simulink model "gm_parallel_lht"  (R2019b)
settings: Solver=FixedStepDiscrete  StartTime=0.0  StopTime=inf  RelTol=1e-3
undefined symbols (not defined in the file or in its folder): bt, height, width
libraries: hdlsllib x190, simulink x13, hdlmdlgenlib x7, dspsrcs4 x1
(part 9 of 18)

== system gm_parallel_lht/Parallel LHT/Parallel LHT Accumulator/Accumulator with Switches/Accumulator_instance1/Block RAM ==
  wr_data : Inport  OutDataTypeStr=fixdt(0, 12, 0)  PortDimensions=1  SampleTime=6.66666666666667e-09
  wr_addr : Inport  Port=2  OutDataTypeStr=fixdt(0, 12, 0)  PortDimensions=1  SampleTime=6.66666666666667e-09
  wr_en : Inport  Port=3  OutDataTypeStr=boolean  PortDimensions=1  SampleTime=6.66666666666667e-09
  rd_addr : Inport  Port=4  OutDataTypeStr=fixdt(0, 12, 0)  PortDimensions=1  SampleTime=6.66666666666667e-09
  Simple Dual Port RAM : Subsystem
  rd_data : Outport
  wires:
  Simple Dual Port RAM/1(rd_data) -> rd_data/1
  wr_data/1 -> Simple Dual Port RAM/1(wr_data)
  wr_addr/1 -> Simple Dual Port RAM/2(wr_addr)
  wr_en/1 -> Simple Dual Port RAM/3(wr_en)
  rd_addr/1 -> Simple Dual Port RAM/4(rd_addr)

== system gm_parallel_lht/Parallel LHT/Parallel LHT Accumulator/Accumulator with Switches/Accumulator_instance10/Block RAM ==
  wr_data : Inport  OutDataTypeStr=fixdt(0, 12, 0)  PortDimensions=1  SampleTime=6.66666666666667e-09
  wr_addr : Inport  Port=2  OutDataTypeStr=fixdt(0, 12, 0)  PortDimensions=1  SampleTime=6.66666666666667e-09
  wr_en : Inport  Port=3  OutDataTypeStr=boolean  PortDimensions=1  SampleTime=6.66666666666667e-09
  rd_addr : Inport  Port=4  OutDataTypeStr=fixdt(0, 12, 0)  PortDimensions=1  SampleTime=6.66666666666667e-09
  Simple Dual Port RAM : Subsystem
  rd_data : Outport
  wires:
  rd_addr/1 -> Simple Dual Port RAM/4(rd_addr)
  wr_en/1 -> Simple Dual Port RAM/3(wr_en)
  wr_addr/1 -> Simple Dual Port RAM/2(wr_addr)
  wr_data/1 -> Simple Dual Port RAM/1(wr_data)
  Simple Dual Port RAM/1(rd_data) -> rd_data/1

== system gm_parallel_lht/Parallel LHT/Parallel LHT Accumulator/Accumulator with Switches/Accumulator_instance100/Block RAM ==
  wr_data : Inport  OutDataTypeStr=fixdt(0, 12, 0)  PortDimensions=1  SampleTime=6.66666666666667e-09
  wr_addr : Inport  Port=2  OutDataTypeStr=fixdt(0, 12, 0)  PortDimensions=1  SampleTime=6.66666666666667e-09
  wr_en : Inport  Port=3  OutDataTypeStr=boolean  PortDimensions=1  SampleTime=6.66666666666667e-09
  rd_addr : Inport  Port=4  OutDataTypeStr=fixdt(0, 12, 0)  PortDimensions=1  SampleTime=6.66666666666667e-09
  Simple Dual Port RAM : Subsystem
  rd_data : Outport
  wires:
  rd_addr/1 -> Simple Dual Port RAM/4(rd_addr)
  wr_en/1 -> Simple Dual Port RAM/3(wr_en)
  wr_addr/1 -> Simple Dual Port RAM/2(wr_addr)
  wr_data/1 -> Simple Dual Port RAM/1(wr_data)
  Simple Dual Port RAM/1(rd_data) -> rd_data/1

== system gm_parallel_lht/Parallel LHT/Parallel LHT Accumulator/Accumulator with Switches/Accumulator_instance101/Block RAM ==
  wr_data : Inport  OutDataTypeStr=fixdt(0, 12, 0)  PortDimensions=1  SampleTime=6.66666666666667e-09
  wr_addr : Inport  Port=2  OutDataTypeStr=fixdt(0, 12, 0)  PortDimensions=1  SampleTime=6.66666666666667e-09
  wr_en : Inport  Port=3  OutDataTypeStr=boolean  PortDimensions=1  SampleTime=6.66666666666667e-09
  rd_addr : Inport  Port=4  OutDataTypeStr=fixdt(0, 12, 0)  PortDimensions=1  SampleTime=6.66666666666667e-09
  Simple Dual Port RAM : Subsystem
  rd_data : Outport
  wires:
  rd_addr/1 -> Simple Dual Port RAM/4(rd_addr)
  wr_en/1 -> Simple Dual Port RAM/3(wr_en)
  wr_addr/1 -> Simple Dual Port RAM/2(wr_addr)
  wr_data/1 -> Simple Dual Port RAM/1(wr_data)
  Simple Dual Port RAM/1(rd_data) -> rd_data/1

== system gm_parallel_lht/Parallel LHT/Parallel LHT Accumulator/Accumulator with Switches/Accumulator_instance102/Block RAM ==
  wr_data : Inport  OutDataTypeStr=fixdt(0, 12, 0)  PortDimensions=1  SampleTime=6.66666666666667e-09
  wr_addr : Inport  Port=2  OutDataTypeStr=fixdt(0, 12, 0)  PortDimensions=1  SampleTime=6.66666666666667e-09
  wr_en : Inport  Port=3  OutDataTypeStr=boolean  PortDimensions=1  SampleTime=6.66666666666667e-09
  rd_addr : Inport  Port=4  OutDataTypeStr=fixdt(0, 12, 0)  PortDimensions=1  SampleTime=6.66666666666667e-09
  Simple Dual Port RAM : Subsystem
  rd_data : Outport
  wires:
  rd_addr/1 -> Simple Dual Port RAM/4(rd_addr)
  wr_en/1 -> Simple Dual Port RAM/3(wr_en)
  wr_addr/1 -> Simple Dual Port RAM/2(wr_addr)
  wr_data/1 -> Simple Dual Port RAM/1(wr_data)
  Simple Dual Port RAM/1(rd_data) -> rd_data/1

== system gm_parallel_lht/Parallel LHT/Parallel LHT Accumulator/Accumulator with Switches/Accumulator_instance103/Block RAM ==
  wr_data : Inport  OutDataTypeStr=fixdt(0, 12, 0)  PortDimensions=1  SampleTime=6.66666666666667e-09
  wr_addr : Inport  Port=2  OutDataTypeStr=fixdt(0, 12, 0)  PortDimensions=1  SampleTime=6.66666666666667e-09
  wr_en : Inport  Port=3  OutDataTypeStr=boolean  PortDimensions=1  SampleTime=6.66666666666667e-09
  rd_addr : Inport  Port=4  OutDataTypeStr=fixdt(0, 12, 0)  PortDimensions=1  SampleTime=6.66666666666667e-09
  Simple Dual Port RAM : Subsystem
  rd_data : Outport
  wires:
  rd_addr/1 -> Simple Dual Port RAM/4(rd_addr)
  wr_en/1 -> Simple Dual Port RAM/3(wr_en)
  wr_addr/1 -> Simple Dual Port RAM/2(wr_addr)
  wr_data/1 -> Simple Dual Port RAM/1(wr_data)
  Simple Dual Port RAM/1(rd_data) -> rd_data/1

== system gm_parallel_lht/Parallel LHT/Parallel LHT Accumulator/Accumulator with Switches/Accumulator_instance104/Block RAM ==
  wr_data : Inport  OutDataTypeStr=fixdt(0, 12, 0)  PortDimensions=1  SampleTime=6.66666666666667e-09
  wr_addr : Inport  Port=2  OutDataTypeStr=fixdt(0, 12, 0)  PortDimensions=1  SampleTime=6.66666666666667e-09
  wr_en : Inport  Port=3  OutDataTypeStr=boolean  PortDimensions=1  SampleTime=6.66666666666667e-09
  rd_addr : Inport  Port=4  OutDataTypeStr=fixdt(0, 12, 0)  PortDimensions=1  SampleTime=6.66666666666667e-09
  Simple Dual Port RAM : Subsystem
  rd_data : Outport
  wires:
  rd_addr/1 -> Simple Dual Port RAM/4(rd_addr)
  wr_en/1 -> Simple Dual Port RAM/3(wr_en)
  wr_addr/1 -> Simple Dual Port RAM/2(wr_addr)
  wr_data/1 -> Simple Dual Port RAM/1(wr_data)
  Simple Dual Port RAM/1(rd_data) -> rd_data/1

== system gm_parallel_lht/Parallel LHT/Parallel LHT Accumulator/Accumulator with Switches/Accumulator_instance105/Block RAM ==
  wr_data : Inport  OutDataTypeStr=fixdt(0, 12, 0)  PortDimensions=1  SampleTime=6.66666666666667e-09
  wr_addr : Inport  Port=2  OutDataTypeStr=fixdt(0, 12, 0)  PortDimensions=1  SampleTime=6.66666666666667e-09
  wr_en : Inport  Port=3  OutDataTypeStr=boolean  PortDimensions=1  SampleTime=6.66666666666667e-09
  rd_addr : Inport  Port=4  OutDataTypeStr=fixdt(0, 12, 0)  PortDimensions=1  SampleTime=6.66666666666667e-09
  Simple Dual Port RAM : Subsystem
  rd_data : Outport
  wires:
  rd_addr/1 -> Simple Dual Port RAM/4(rd_addr)
  wr_en/1 -> Simple Dual Port RAM/3(wr_en)
  wr_addr/1 -> Simple Dual Port RAM/2(wr_addr)
  wr_data/1 -> Simple Dual Port RAM/1(wr_data)
  Simple Dual Port RAM/1(rd_data) -> rd_data/1

== system gm_parallel_lht/Parallel LHT/Parallel LHT Accumulator/Accumulator with Switches/Accumulator_instance106/Block RAM ==
  wr_data : Inport  OutDataTypeStr=fixdt(0, 12, 0)  PortDimensions=1  SampleTime=6.66666666666667e-09
  wr_addr : Inport  Port=2  OutDataTypeStr=fixdt(0, 12, 0)  PortDimensions=1  SampleTime=6.66666666666667e-09
  wr_en : Inport  Port=3  OutDataTypeStr=boolean  PortDimensions=1  SampleTime=6.66666666666667e-09
  rd_addr : Inport  Port=4  OutDataTypeStr=fixdt(0, 12, 0)  PortDimensions=1  SampleTime=6.66666666666667e-09
  Simple Dual Port RAM : Subsystem
  rd_data : Outport
  wires:
  rd_addr/1 -> Simple Dual Port RAM/4(rd_addr)
  wr_en/1 -> Simple Dual Port RAM/3(wr_en)
  wr_addr/1 -> Simple Dual Port RAM/2(wr_addr)
  wr_data/1 -> Simple Dual Port RAM/1(wr_data)
  Simple Dual Port RAM/1(rd_data) -> rd_data/1

== system gm_parallel_lht/Parallel LHT/Parallel LHT Accumulator/Accumulator with Switches/Accumulator_instance107/Block RAM ==
  wr_data : Inport  OutDataTypeStr=fixdt(0, 12, 0)  PortDimensions=1  SampleTime=6.66666666666667e-09
  wr_addr : Inport  Port=2  OutDataTypeStr=fixdt(0, 12, 0)  PortDimensions=1  SampleTime=6.66666666666667e-09
  wr_en : Inport  Port=3  OutDataTypeStr=boolean  PortDimensions=1  SampleTime=6.66666666666667e-09
  rd_addr : Inport  Port=4  OutDataTypeStr=fixdt(0, 12, 0)  PortDimensions=1  SampleTime=6.66666666666667e-09
  Simple Dual Port RAM : Subsystem
  rd_data : Outport
  wires:
  rd_addr/1 -> Simple Dual Port RAM/4(rd_addr)
  wr_en/1 -> Simple Dual Port RAM/3(wr_en)
  wr_addr/1 -> Simple Dual Port RAM/2(wr_addr)
  wr_data/1 -> Simple Dual Port RAM/1(wr_data)
  Simple Dual Port RAM/1(rd_data) -> rd_data/1

== system gm_parallel_lht/Parallel LHT/Parallel LHT Accumulator/Accumulator with Switches/Accumulator_instance108/Block RAM ==
  wr_data : Inport  OutDataTypeStr=fixdt(0, 12, 0)  PortDimensions=1  SampleTime=6.66666666666667e-09
  wr_addr : Inport  Port=2  OutDataTypeStr=fixdt(0, 12, 0)  PortDimensions=1  SampleTime=6.66666666666667e-09
  wr_en : Inport  Port=3  OutDataTypeStr=boolean  PortDimensions=1  SampleTime=6.66666666666667e-09
  rd_addr : Inport  Port=4  OutDataTypeStr=fixdt(0, 12, 0)  PortDimensions=1  SampleTime=6.66666666666667e-09
  Simple Dual Port RAM : Subsystem
  rd_data : Outport
  wires:
  rd_addr/1 -> Simple Dual Port RAM/4(rd_addr)
  wr_en/1 -> Simple Dual Port RAM/3(wr_en)
  wr_addr/1 -> Simple Dual Port RAM/2(wr_addr)
  wr_data/1 -> Simple Dual Port RAM/1(wr_data)
  Simple Dual Port RAM/1(rd_data) -> rd_data/1

== system gm_parallel_lht/Parallel LHT/Parallel LHT Accumulator/Accumulator with Switches/Accumulator_instance109/Block RAM ==
  wr_data : Inport  OutDataTypeStr=fixdt(0, 12, 0)  PortDimensions=1  SampleTime=6.66666666666667e-09
  wr_addr : Inport  Port=2  OutDataTypeStr=fixdt(0, 12, 0)  PortDimensions=1  SampleTime=6.66666666666667e-09
  wr_en : Inport  Port=3  OutDataTypeStr=boolean  PortDimensions=1  SampleTime=6.66666666666667e-09
  rd_addr : Inport  Port=4  OutDataTypeStr=fixdt(0, 12, 0)  PortDimensions=1  SampleTime=6.66666666666667e-09
  Simple Dual Port RAM : Subsystem
  rd_data : Outport
  wires:
  rd_addr/1 -> Simple Dual Port RAM/4(rd_addr)
  wr_en/1 -> Simple Dual Port RAM/3(wr_en)
  wr_addr/1 -> Simple Dual Port RAM/2(wr_addr)
  wr_data/1 -> Simple Dual Port RAM/1(wr_data)
  Simple Dual Port RAM/1(rd_data) -> rd_data/1

== system gm_parallel_lht/Parallel LHT/Parallel LHT Accumulator/Accumulator with Switches/Accumulator_instance11/Block RAM ==
  wr_data : Inport  OutDataTypeStr=fixdt(0, 12, 0)  PortDimensions=1  SampleTime=6.66666666666667e-09
  wr_addr : Inport  Port=2  OutDataTypeStr=fixdt(0, 12, 0)  PortDimensions=1  SampleTime=6.66666666666667e-09
  wr_en : Inport  Port=3  OutDataTypeStr=boolean  PortDimensions=1  SampleTime=6.66666666666667e-09
  rd_addr : Inport  Port=4  OutDataTypeStr=fixdt(0, 12, 0)  PortDimensions=1  SampleTime=6.66666666666667e-09
  Simple Dual Port RAM : Subsystem
  rd_data : Outport
  wires:
  rd_addr/1 -> Simple Dual Port RAM/4(rd_addr)
  wr_en/1 -> Simple Dual Port RAM/3(wr_en)
  wr_addr/1 -> Simple Dual Port RAM/2(wr_addr)
  wr_data/1 -> Simple Dual Port RAM/1(wr_data)
  Simple Dual Port RAM/1(rd_data) -> rd_data/1

== system gm_parallel_lht/Parallel LHT/Parallel LHT Accumulator/Accumulator with Switches/Accumulator_instance110/Block RAM ==
  wr_data : Inport  OutDataTypeStr=fixdt(0, 12, 0)  PortDimensions=1  SampleTime=6.66666666666667e-09
  wr_addr : Inport  Port=2  OutDataTypeStr=fixdt(0, 12, 0)  PortDimensions=1  SampleTime=6.66666666666667e-09
  wr_en : Inport  Port=3  OutDataTypeStr=boolean  PortDimensions=1  SampleTime=6.66666666666667e-09
  rd_addr : Inport  Port=4  OutDataTypeStr=fixdt(0, 12, 0)  PortDimensions=1  SampleTime=6.66666666666667e-09
  Simple Dual Port RAM : Subsystem
  rd_data : Outport
  wires:
  rd_addr/1 -> Simple Dual Port RAM/4(rd_addr)
  wr_en/1 -> Simple Dual Port RAM/3(wr_en)
  wr_addr/1 -> Simple Dual Port RAM/2(wr_addr)
  wr_data/1 -> Simple Dual Port RAM/1(wr_data)
  Simple Dual Port RAM/1(rd_data) -> rd_data/1

== system gm_parallel_lht/Parallel LHT/Parallel LHT Accumulator/Accumulator with Switches/Accumulator_instance111/Block RAM ==
  wr_data : Inport  OutDataTypeStr=fixdt(0, 12, 0)  PortDimensions=1  SampleTime=6.66666666666667e-09
  wr_addr : Inport  Port=2  OutDataTypeStr=fixdt(0, 12, 0)  PortDimensions=1  SampleTime=6.66666666666667e-09
  wr_en : Inport  Port=3  OutDataTypeStr=boolean  PortDimensions=1  SampleTime=6.66666666666667e-09
  rd_addr : Inport  Port=4  OutDataTypeStr=fixdt(0, 12, 0)  PortDimensions=1  SampleTime=6.66666666666667e-09
  Simple Dual Port RAM : Subsystem
  rd_data : Outport
  wires:
  rd_addr/1 -> Simple Dual Port RAM/4(rd_addr)
  wr_en/1 -> Simple Dual Port RAM/3(wr_en)
  wr_addr/1 -> Simple Dual Port RAM/2(wr_addr)
  wr_data/1 -> Simple Dual Port RAM/1(wr_data)
  Simple Dual Port RAM/1(rd_data) -> rd_data/1

== system gm_parallel_lht/Parallel LHT/Parallel LHT Accumulator/Accumulator with Switches/Accumulator_instance112/Block RAM ==
  wr_data : Inport  OutDataTypeStr=fixdt(0, 12, 0)  PortDimensions=1  SampleTime=6.66666666666667e-09
  wr_addr : Inport  Port=2  OutDataTypeStr=fixdt(0, 12, 0)  PortDimensions=1  SampleTime=6.66666666666667e-09
  wr_en : Inport  Port=3  OutDataTypeStr=boolean  PortDimensions=1  SampleTime=6.66666666666667e-09
  rd_addr : Inport  Port=4  OutDataTypeStr=fixdt(0, 12, 0)  PortDimensions=1  SampleTime=6.66666666666667e-09
  Simple Dual Port RAM : Subsystem
  rd_data : Outport
  wires:
  rd_addr/1 -> Simple Dual Port RAM/4(rd_addr)
  wr_en/1 -> Simple Dual Port RAM/3(wr_en)
  wr_addr/1 -> Simple Dual Port RAM/2(wr_addr)
  wr_data/1 -> Simple Dual Port RAM/1(wr_data)
  Simple Dual Port RAM/1(rd_data) -> rd_data/1

== system gm_parallel_lht/Parallel LHT/Parallel LHT Accumulator/Accumulator with Switches/Accumulator_instance113/Block RAM ==
  wr_data : Inport  OutDataTypeStr=fixdt(0, 12, 0)  PortDimensions=1  SampleTime=6.66666666666667e-09
  wr_addr : Inport  Port=2  OutDataTypeStr=fixdt(0, 12, 0)  PortDimensions=1  SampleTime=6.66666666666667e-09
  wr_en : Inport  Port=3  OutDataTypeStr=boolean  PortDimensions=1  SampleTime=6.66666666666667e-09
  rd_addr : Inport  Port=4  OutDataTypeStr=fixdt(0, 12, 0)  PortDimensions=1  SampleTime=6.66666666666667e-09
  Simple Dual Port RAM : Subsystem
  rd_data : Outport
  wires:
  rd_addr/1 -> Simple Dual Port RAM/4(rd_addr)
  wr_en/1 -> Simple Dual Port RAM/3(wr_en)
  wr_addr/1 -> Simple Dual Port RAM/2(wr_addr)
  wr_data/1 -> Simple Dual Port RAM/1(wr_data)
  Simple Dual Port RAM/1(rd_data) -> rd_data/1

== system gm_parallel_lht/Parallel LHT/Parallel LHT Accumulator/Accumulator with Switches/Accumulator_instance114/Block RAM ==
  wr_data : Inport  OutDataTypeStr=fixdt(0, 12, 0)  PortDimensions=1  SampleTime=6.66666666666667e-09
  wr_addr : Inport  Port=2  OutDataTypeStr=fixdt(0, 12, 0)  PortDimensions=1  SampleTime=6.66666666666667e-09
  wr_en : Inport  Port=3  OutDataTypeStr=boolean  PortDimensions=1  SampleTime=6.66666666666667e-09
  rd_addr : Inport  Port=4  OutDataTypeStr=fixdt(0, 12, 0)  PortDimensions=1  SampleTime=6.66666666666667e-09
  Simple Dual Port RAM : Subsystem
  rd_data : Outport
  wires:
  rd_addr/1 -> Simple Dual Port RAM/4(rd_addr)
  wr_en/1 -> Simple Dual Port RAM/3(wr_en)
  wr_addr/1 -> Simple Dual Port RAM/2(wr_addr)
  wr_data/1 -> Simple Dual Port RAM/1(wr_data)
  Simple Dual Port RAM/1(rd_data) -> rd_data/1

== system gm_parallel_lht/Parallel LHT/Parallel LHT Accumulator/Accumulator with Switches/Accumulator_instance115/Block RAM ==
  wr_data : Inport  OutDataTypeStr=fixdt(0, 12, 0)  PortDimensions=1  SampleTime=6.66666666666667e-09
  wr_addr : Inport  Port=2  OutDataTypeStr=fixdt(0, 12, 0)  PortDimensions=1  SampleTime=6.66666666666667e-09
  wr_en : Inport  Port=3  OutDataTypeStr=boolean  PortDimensions=1  SampleTime=6.66666666666667e-09
  rd_addr : Inport  Port=4  OutDataTypeStr=fixdt(0, 12, 0)  PortDimensions=1  SampleTime=6.66666666666667e-09
  Simple Dual Port RAM : Subsystem
  rd_data : Outport
  wires:
  rd_addr/1 -> Simple Dual Port RAM/4(rd_addr)
  wr_en/1 -> Simple Dual Port RAM/3(wr_en)
  wr_addr/1 -> Simple Dual Port RAM/2(wr_addr)
  wr_data/1 -> Simple Dual Port RAM/1(wr_data)
  Simple Dual Port RAM/1(rd_data) -> rd_data/1

== system gm_parallel_lht/Parallel LHT/Parallel LHT Accumulator/Accumulator with Switches/Accumulator_instance116/Block RAM ==
  wr_data : Inport  OutDataTypeStr=fixdt(0, 12, 0)  PortDimensions=1  SampleTime=6.66666666666667e-09
  wr_addr : Inport  Port=2  OutDataTypeStr=fixdt(0, 12, 0)  PortDimensions=1  SampleTime=6.66666666666667e-09
  wr_en : Inport  Port=3  OutDataTypeStr=boolean  PortDimensions=1  SampleTime=6.66666666666667e-09
  rd_addr : Inport  Port=4  OutDataTypeStr=fixdt(0, 12, 0)  PortDimensions=1  SampleTime=6.66666666666667e-09
  Simple Dual Port RAM : Subsystem
  rd_data : Outport
  wires:
  rd_addr/1 -> Simple Dual Port RAM/4(rd_addr)
  wr_en/1 -> Simple Dual Port RAM/3(wr_en)
  wr_addr/1 -> Simple Dual Port RAM/2(wr_addr)
  wr_data/1 -> Simple Dual Port RAM/1(wr_data)
  Simple Dual Port RAM/1(rd_data) -> rd_data/1

== system gm_parallel_lht/Parallel LHT/Parallel LHT Accumulator/Accumulator with Switches/Accumulator_instance117/Block RAM ==
  wr_data : Inport  OutDataTypeStr=fixdt(0, 12, 0)  PortDimensions=1  SampleTime=6.66666666666667e-09
  wr_addr : Inport  Port=2  OutDataTypeStr=fixdt(0, 12, 0)  PortDimensions=1  SampleTime=6.66666666666667e-09
  wr_en : Inport  Port=3  OutDataTypeStr=boolean  PortDimensions=1  SampleTime=6.66666666666667e-09
  rd_addr : Inport  Port=4  OutDataTypeStr=fixdt(0, 12, 0)  PortDimensions=1  SampleTime=6.66666666666667e-09
  Simple Dual Port RAM : Subsystem
  rd_data : Outport
  wires:
  rd_addr/1 -> Simple Dual Port RAM/4(rd_addr)
  wr_en/1 -> Simple Dual Port RAM/3(wr_en)
  wr_addr/1 -> Simple Dual Port RAM/2(wr_addr)
  wr_data/1 -> Simple Dual Port RAM/1(wr_data)
  Simple Dual Port RAM/1(rd_data) -> rd_data/1

== system gm_parallel_lht/Parallel LHT/Parallel LHT Accumulator/Accumulator with Switches/Accumulator_instance118/Block RAM ==
  wr_data : Inport  OutDataTypeStr=fixdt(0, 12, 0)  PortDimensions=1  SampleTime=6.66666666666667e-09
  wr_addr : Inport  Port=2  OutDataTypeStr=fixdt(0, 12, 0)  PortDimensions=1  SampleTime=6.66666666666667e-09
  wr_en : Inport  Port=3  OutDataTypeStr=boolean  PortDimensions=1  SampleTime=6.66666666666667e-09
  rd_addr : Inport  Port=4  OutDataTypeStr=fixdt(0, 12, 0)  PortDimensions=1  SampleTime=6.66666666666667e-09
  Simple Dual Port RAM : Subsystem
  rd_data : Outport
  wires:
  rd_addr/1 -> Simple Dual Port RAM/4(rd_addr)
  wr_en/1 -> Simple Dual Port RAM/3(wr_en)
  wr_addr/1 -> Simple Dual Port RAM/2(wr_addr)
  wr_data/1 -> Simple Dual Port RAM/1(wr_data)
  Simple Dual Port RAM/1(rd_data) -> rd_data/1

== system gm_parallel_lht/Parallel LHT/Parallel LHT Accumulator/Accumulator with Switches/Accumulator_instance119/Block RAM ==
  wr_data : Inport  OutDataTypeStr=fixdt(0, 12, 0)  PortDimensions=1  SampleTime=6.66666666666667e-09
  wr_addr : Inport  Port=2  OutDataTypeStr=fixdt(0, 12, 0)  PortDimensions=1  SampleTime=6.66666666666667e-09
  wr_en : Inport  Port=3  OutDataTypeStr=boolean  PortDimensions=1  SampleTime=6.66666666666667e-09
  rd_addr : Inport  Port=4  OutDataTypeStr=fixdt(0, 12, 0)  PortDimensions=1  SampleTime=6.66666666666667e-09
  Simple Dual Port RAM : Subsystem
  rd_data : Outport
  wires:
  rd_addr/1 -> Simple Dual Port RAM/4(rd_addr)
  wr_en/1 -> Simple Dual Port RAM/3(wr_en)
  wr_addr/1 -> Simple Dual Port RAM/2(wr_addr)
  wr_data/1 -> Simple Dual Port RAM/1(wr_data)
  Simple Dual Port RAM/1(rd_data) -> rd_data/1

== system gm_parallel_lht/Parallel LHT/Parallel LHT Accumulator/Accumulator with Switches/Accumulator_instance12/Block RAM ==
  wr_data : Inport  OutDataTypeStr=fixdt(0, 12, 0)  PortDimensions=1  SampleTime=6.66666666666667e-09
  wr_addr : Inport  Port=2  OutDataTypeStr=fixdt(0, 12, 0)  PortDimensions=1  SampleTime=6.66666666666667e-09
  wr_en : Inport  Port=3  OutDataTypeStr=boolean  PortDimensions=1  SampleTime=6.66666666666667e-09
  rd_addr : Inport  Port=4  OutDataTypeStr=fixdt(0, 12, 0)  PortDimensions=1  SampleTime=6.66666666666667e-09
  Simple Dual Port RAM : Subsystem
  rd_data : Outport
  wires:
  rd_addr/1 -> Simple Dual Port RAM/4(rd_addr)
  wr_en/1 -> Simple Dual Port RAM/3(wr_en)
  wr_addr/1 -> Simple Dual Port RAM/2(wr_addr)
  wr_data/1 -> Simple Dual Port RAM/1(wr_data)
  Simple Dual Port RAM/1(rd_data) -> rd_data/1

== system gm_parallel_lht/Parallel LHT/Parallel LHT Accumulator/Accumulator with Switches/Accumulator_instance120/Block RAM ==
  wr_data : Inport  OutDataTypeStr=fixdt(0, 12, 0)  PortDimensions=1  SampleTime=6.66666666666667e-09
  wr_addr : Inport  Port=2  OutDataTypeStr=fixdt(0, 12, 0)  PortDimensions=1  SampleTime=6.66666666666667e-09
  wr_en : Inport  Port=3  OutDataTypeStr=boolean  PortDimensions=1  SampleTime=6.66666666666667e-09
  rd_addr : Inport  Port=4  OutDataTypeStr=fixdt(0, 12, 0)  PortDimensions=1  SampleTime=6.66666666666667e-09
  Simple Dual Port RAM : Subsystem
  rd_data : Outport
  wires:
  rd_addr/1 -> Simple Dual Port RAM/4(rd_addr)
  wr_en/1 -> Simple Dual Port RAM/3(wr_en)
  wr_addr/1 -> Simple Dual Port RAM/2(wr_addr)
  wr_data/1 -> Simple Dual Port RAM/1(wr_data)
  Simple Dual Port RAM/1(rd_data) -> rd_data/1

== system gm_parallel_lht/Parallel LHT/Parallel LHT Accumulator/Accumulator with Switches/Accumulator_instance121/Block RAM ==
  wr_data : Inport  OutDataTypeStr=fixdt(0, 12, 0)  PortDimensions=1  SampleTime=6.66666666666667e-09
  wr_addr : Inport  Port=2  OutDataTypeStr=fixdt(0, 12, 0)  PortDimensions=1  SampleTime=6.66666666666667e-09
  wr_en : Inport  Port=3  OutDataTypeStr=boolean  PortDimensions=1  SampleTime=6.66666666666667e-09
  rd_addr : Inport  Port=4  OutDataTypeStr=fixdt(0, 12, 0)  PortDimensions=1  SampleTime=6.66666666666667e-09
  Simple Dual Port RAM : Subsystem
  rd_data : Outport
  wires:
  rd_addr/1 -> Simple Dual Port RAM/4(rd_addr)
  wr_en/1 -> Simple Dual Port RAM/3(wr_en)
  wr_addr/1 -> Simple Dual Port RAM/2(wr_addr)
  wr_data/1 -> Simple Dual Port RAM/1(wr_data)
  Simple Dual Port RAM/1(rd_data) -> rd_data/1

== system gm_parallel_lht/Parallel LHT/Parallel LHT Accumulator/Accumulator with Switches/Accumulator_instance122/Block RAM ==
  wr_data : Inport  OutDataTypeStr=fixdt(0, 12, 0)  PortDimensions=1  SampleTime=6.66666666666667e-09
  wr_addr : Inport  Port=2  OutDataTypeStr=fixdt(0, 12, 0)  PortDimensions=1  SampleTime=6.66666666666667e-09
  wr_en : Inport  Port=3  OutDataTypeStr=boolean  PortDimensions=1  SampleTime=6.66666666666667e-09
  rd_addr : Inport  Port=4  OutDataTypeStr=fixdt(0, 12, 0)  PortDimensions=1  SampleTime=6.66666666666667e-09
  Simple Dual Port RAM : Subsystem
  rd_data : Outport
  wires:
  rd_addr/1 -> Simple Dual Port RAM/4(rd_addr)
  wr_en/1 -> Simple Dual Port RAM/3(wr_en)
  wr_addr/1 -> Simple Dual Port RAM/2(wr_addr)
  wr_data/1 -> Simple Dual Port RAM/1(wr_data)
  Simple Dual Port RAM/1(rd_data) -> rd_data/1

== system gm_parallel_lht/Parallel LHT/Parallel LHT Accumulator/Accumulator with Switches/Accumulator_instance123/Block RAM ==
  wr_data : Inport  OutDataTypeStr=fixdt(0, 12, 0)  PortDimensions=1  SampleTime=6.66666666666667e-09
  wr_addr : Inport  Port=2  OutDataTypeStr=fixdt(0, 12, 0)  PortDimensions=1  SampleTime=6.66666666666667e-09
  wr_en : Inport  Port=3  OutDataTypeStr=boolean  PortDimensions=1  SampleTime=6.66666666666667e-09
  rd_addr : Inport  Port=4  OutDataTypeStr=fixdt(0, 12, 0)  PortDimensions=1  SampleTime=6.66666666666667e-09
  Simple Dual Port RAM : Subsystem
  rd_data : Outport
  wires:
  rd_addr/1 -> Simple Dual Port RAM/4(rd_addr)
  wr_en/1 -> Simple Dual Port RAM/3(wr_en)
  wr_addr/1 -> Simple Dual Port RAM/2(wr_addr)
  wr_data/1 -> Simple Dual Port RAM/1(wr_data)
  Simple Dual Port RAM/1(rd_data) -> rd_data/1

== system gm_parallel_lht/Parallel LHT/Parallel LHT Accumulator/Accumulator with Switches/Accumulator_instance124/Block RAM ==
  wr_data : Inport  OutDataTypeStr=fixdt(0, 12, 0)  PortDimensions=1  SampleTime=6.66666666666667e-09
  wr_addr : Inport  Port=2  OutDataTypeStr=fixdt(0, 12, 0)  PortDimensions=1  SampleTime=6.66666666666667e-09
  wr_en : Inport  Port=3  OutDataTypeStr=boolean  PortDimensions=1  SampleTime=6.66666666666667e-09
  rd_addr : Inport  Port=4  OutDataTypeStr=fixdt(0, 12, 0)  PortDimensions=1  SampleTime=6.66666666666667e-09
  Simple Dual Port RAM : Subsystem
  rd_data : Outport
  wires:
  rd_addr/1 -> Simple Dual Port RAM/4(rd_addr)
  wr_en/1 -> Simple Dual Port RAM/3(wr_en)
  wr_addr/1 -> Simple Dual Port RAM/2(wr_addr)
  wr_data/1 -> Simple Dual Port RAM/1(wr_data)
  Simple Dual Port RAM/1(rd_data) -> rd_data/1

== system gm_parallel_lht/Parallel LHT/Parallel LHT Accumulator/Accumulator with Switches/Accumulator_instance125/Block RAM ==
  wr_data : Inport  OutDataTypeStr=fixdt(0, 12, 0)  PortDimensions=1  SampleTime=6.66666666666667e-09
  wr_addr : Inport  Port=2  OutDataTypeStr=fixdt(0, 12, 0)  PortDimensions=1  SampleTime=6.66666666666667e-09
  wr_en : Inport  Port=3  OutDataTypeStr=boolean  PortDimensions=1  SampleTime=6.66666666666667e-09
  rd_addr : Inport  Port=4  OutDataTypeStr=fixdt(0, 12, 0)  PortDimensions=1  SampleTime=6.66666666666667e-09
  Simple Dual Port RAM : Subsystem
  rd_data : Outport
  wires:
  rd_addr/1 -> Simple Dual Port RAM/4(rd_addr)
  wr_en/1 -> Simple Dual Port RAM/3(wr_en)
  wr_addr/1 -> Simple Dual Port RAM/2(wr_addr)
  wr_data/1 -> Simple Dual Port RAM/1(wr_data)
  Simple Dual Port RAM/1(rd_data) -> rd_data/1

== system gm_parallel_lht/Parallel LHT/Parallel LHT Accumulator/Accumulator with Switches/Accumulator_instance126/Block RAM ==
  wr_data : Inport  OutDataTypeStr=fixdt(0, 12, 0)  PortDimensions=1  SampleTime=6.66666666666667e-09
  wr_addr : Inport  Port=2  OutDataTypeStr=fixdt(0, 12, 0)  PortDimensions=1  SampleTime=6.66666666666667e-09
  wr_en : Inport  Port=3  OutDataTypeStr=boolean  PortDimensions=1  SampleTime=6.66666666666667e-09
  rd_addr : Inport  Port=4  OutDataTypeStr=fixdt(0, 12, 0)  PortDimensions=1  SampleTime=6.66666666666667e-09
  Simple Dual Port RAM : Subsystem
  rd_data : Outport
  wires:
  rd_addr/1 -> Simple Dual Port RAM/4(rd_addr)
  wr_en/1 -> Simple Dual Port RAM/3(wr_en)
  wr_addr/1 -> Simple Dual Port RAM/2(wr_addr)
  wr_data/1 -> Simple Dual Port RAM/1(wr_data)
  Simple Dual Port RAM/1(rd_data) -> rd_data/1

== system gm_parallel_lht/Parallel LHT/Parallel LHT Accumulator/Accumulator with Switches/Accumulator_instance127/Block RAM ==
  wr_data : Inport  OutDataTypeStr=fixdt(0, 12, 0)  PortDimensions=1  SampleTime=6.66666666666667e-09
  wr_addr : Inport  Port=2  OutDataTypeStr=fixdt(0, 12, 0)  PortDimensions=1  SampleTime=6.66666666666667e-09
  wr_en : Inport  Port=3  OutDataTypeStr=boolean  PortDimensions=1  SampleTime=6.66666666666667e-09
  rd_addr : Inport  Port=4  OutDataTypeStr=fixdt(0, 12, 0)  PortDimensions=1  SampleTime=6.66666666666667e-09
  Simple Dual Port RAM : Subsystem
  rd_data : Outport
  wires:
  rd_addr/1 -> Simple Dual Port RAM/4(rd_addr)
  wr_en/1 -> Simple Dual Port RAM/3(wr_en)
  wr_addr/1 -> Simple Dual Port RAM/2(wr_addr)
  wr_data/1 -> Simple Dual Port RAM/1(wr_data)
  Simple Dual Port RAM/1(rd_data) -> rd_data/1

== system gm_parallel_lht/Parallel LHT/Parallel LHT Accumulator/Accumulator with Switches/Accumulator_instance128/Block RAM ==
  wr_data : Inport  OutDataTypeStr=fixdt(0, 12, 0)  PortDimensions=1  SampleTime=6.66666666666667e-09
  wr_addr : Inport  Port=2  OutDataTypeStr=fixdt(0, 12, 0)  PortDimensions=1  SampleTime=6.66666666666667e-09
  wr_en : Inport  Port=3  OutDataTypeStr=boolean  PortDimensions=1  SampleTime=6.66666666666667e-09
  rd_addr : Inport  Port=4  OutDataTypeStr=fixdt(0, 12, 0)  PortDimensions=1  SampleTime=6.66666666666667e-09
  Simple Dual Port RAM : Subsystem
  rd_data : Outport
  wires:
  rd_addr/1 -> Simple Dual Port RAM/4(rd_addr)
  wr_en/1 -> Simple Dual Port RAM/3(wr_en)
  wr_addr/1 -> Simple Dual Port RAM/2(wr_addr)
  wr_data/1 -> Simple Dual Port RAM/1(wr_data)
  Simple Dual Port RAM/1(rd_data) -> rd_data/1

== system gm_parallel_lht/Parallel LHT/Parallel LHT Accumulator/Accumulator with Switches/Accumulator_instance129/Block RAM ==
  wr_data : Inport  OutDataTypeStr=fixdt(0, 12, 0)  PortDimensions=1  SampleTime=6.66666666666667e-09
  wr_addr : Inport  Port=2  OutDataTypeStr=fixdt(0, 12, 0)  PortDimensions=1  SampleTime=6.66666666666667e-09
  wr_en : Inport  Port=3  OutDataTypeStr=boolean  PortDimensions=1  SampleTime=6.66666666666667e-09
  rd_addr : Inport  Port=4  OutDataTypeStr=fixdt(0, 12, 0)  PortDimensions=1  SampleTime=6.66666666666667e-09
  Simple Dual Port RAM : Subsystem
  rd_data : Outport
  wires:
  rd_addr/1 -> Simple Dual Port RAM/4(rd_addr)
  wr_en/1 -> Simple Dual Port RAM/3(wr_en)
  wr_addr/1 -> Simple Dual Port RAM/2(wr_addr)
  wr_data/1 -> Simple Dual Port RAM/1(wr_data)
  Simple Dual Port RAM/1(rd_data) -> rd_data/1

== system gm_parallel_lht/Parallel LHT/Parallel LHT Accumulator/Accumulator with Switches/Accumulator_instance13/Block RAM ==
  wr_data : Inport  OutDataTypeStr=fixdt(0, 12, 0)  PortDimensions=1  SampleTime=6.66666666666667e-09
  wr_addr : Inport  Port=2  OutDataTypeStr=fixdt(0, 12, 0)  PortDimensions=1  SampleTime=6.66666666666667e-09
  wr_en : Inport  Port=3  OutDataTypeStr=boolean  PortDimensions=1  SampleTime=6.66666666666667e-09
  rd_addr : Inport  Port=4  OutDataTypeStr=fixdt(0, 12, 0)  PortDimensions=1  SampleTime=6.66666666666667e-09
  Simple Dual Port RAM : Subsystem
  rd_data : Outport
  wires:
  rd_addr/1 -> Simple Dual Port RAM/4(rd_addr)
  wr_en/1 -> Simple Dual Port RAM/3(wr_en)
  wr_addr/1 -> Simple Dual Port RAM/2(wr_addr)
  wr_data/1 -> Simple Dual Port RAM/1(wr_data)
  Simple Dual Port RAM/1(rd_data) -> rd_data/1

== system gm_parallel_lht/Parallel LHT/Parallel LHT Accumulator/Accumulator with Switches/Accumulator_instance130/Block RAM ==
  wr_data : Inport  OutDataTypeStr=fixdt(0, 12, 0)  PortDimensions=1  SampleTime=6.66666666666667e-09
  wr_addr : Inport  Port=2  OutDataTypeStr=fixdt(0, 12, 0)  PortDimensions=1  SampleTime=6.66666666666667e-09
  wr_en : Inport  Port=3  OutDataTypeStr=boolean  PortDimensions=1  SampleTime=6.66666666666667e-09
  rd_addr : Inport  Port=4  OutDataTypeStr=fixdt(0, 12, 0)  PortDimensions=1  SampleTime=6.66666666666667e-09
  Simple Dual Port RAM : Subsystem
  rd_data : Outport
  wires:
  rd_addr/1 -> Simple Dual Port RAM/4(rd_addr)
  wr_en/1 -> Simple Dual Port RAM/3(wr_en)
  wr_addr/1 -> Simple Dual Port RAM/2(wr_addr)
  wr_data/1 -> Simple Dual Port RAM/1(wr_data)
  Simple Dual Port RAM/1(rd_data) -> rd_data/1

== system gm_parallel_lht/Parallel LHT/Parallel LHT Accumulator/Accumulator with Switches/Accumulator_instance131/Block RAM ==
  wr_data : Inport  OutDataTypeStr=fixdt(0, 12, 0)  PortDimensions=1  SampleTime=6.66666666666667e-09
  wr_addr : Inport  Port=2  OutDataTypeStr=fixdt(0, 12, 0)  PortDimensions=1  SampleTime=6.66666666666667e-09
  wr_en : Inport  Port=3  OutDataTypeStr=boolean  PortDimensions=1  SampleTime=6.66666666666667e-09
  rd_addr : Inport  Port=4  OutDataTypeStr=fixdt(0, 12, 0)  PortDimensions=1  SampleTime=6.66666666666667e-09
  Simple Dual Port RAM : Subsystem
  rd_data : Outport
  wires:
  rd_addr/1 -> Simple Dual Port RAM/4(rd_addr)
  wr_en/1 -> Simple Dual Port RAM/3(wr_en)
  wr_addr/1 -> Simple Dual Port RAM/2(wr_addr)
  wr_data/1 -> Simple Dual Port RAM/1(wr_data)
  Simple Dual Port RAM/1(rd_data) -> rd_data/1

== system gm_parallel_lht/Parallel LHT/Parallel LHT Accumulator/Accumulator with Switches/Accumulator_instance132/Block RAM ==
  wr_data : Inport  OutDataTypeStr=fixdt(0, 12, 0)  PortDimensions=1  SampleTime=6.66666666666667e-09
  wr_addr : Inport  Port=2  OutDataTypeStr=fixdt(0, 12, 0)  PortDimensions=1  SampleTime=6.66666666666667e-09
  wr_en : Inport  Port=3  OutDataTypeStr=boolean  PortDimensions=1  SampleTime=6.66666666666667e-09
  rd_addr : Inport  Port=4  OutDataTypeStr=fixdt(0, 12, 0)  PortDimensions=1  SampleTime=6.66666666666667e-09
  Simple Dual Port RAM : Subsystem
  rd_data : Outport
  wires:
  rd_addr/1 -> Simple Dual Port RAM/4(rd_addr)
  wr_en/1 -> Simple Dual Port RAM/3(wr_en)
  wr_addr/1 -> Simple Dual Port RAM/2(wr_addr)
  wr_data/1 -> Simple Dual Port RAM/1(wr_data)
  Simple Dual Port RAM/1(rd_data) -> rd_data/1

== system gm_parallel_lht/Parallel LHT/Parallel LHT Accumulator/Accumulator with Switches/Accumulator_instance133/Block RAM ==
  wr_data : Inport  OutDataTypeStr=fixdt(0, 12, 0)  PortDimensions=1  SampleTime=6.66666666666667e-09
  wr_addr : Inport  Port=2  OutDataTypeStr=fixdt(0, 12, 0)  PortDimensions=1  SampleTime=6.66666666666667e-09
  wr_en : Inport  Port=3  OutDataTypeStr=boolean  PortDimensions=1  SampleTime=6.66666666666667e-09
  rd_addr : Inport  Port=4  OutDataTypeStr=fixdt(0, 12, 0)  PortDimensions=1  SampleTime=6.66666666666667e-09
  Simple Dual Port RAM : Subsystem
  rd_data : Outport
  wires:
  rd_addr/1 -> Simple Dual Port RAM/4(rd_addr)
  wr_en/1 -> Simple Dual Port RAM/3(wr_en)
  wr_addr/1 -> Simple Dual Port RAM/2(wr_addr)
  wr_data/1 -> Simple Dual Port RAM/1(wr_data)
  Simple Dual Port RAM/1(rd_data) -> rd_data/1

== system gm_parallel_lht/Parallel LHT/Parallel LHT Accumulator/Accumulator with Switches/Accumulator_instance134/Block RAM ==
  wr_data : Inport  OutDataTypeStr=fixdt(0, 12, 0)  PortDimensions=1  SampleTime=6.66666666666667e-09
  wr_addr : Inport  Port=2  OutDataTypeStr=fixdt(0, 12, 0)  PortDimensions=1  SampleTime=6.66666666666667e-09
  wr_en : Inport  Port=3  OutDataTypeStr=boolean  PortDimensions=1  SampleTime=6.66666666666667e-09
  rd_addr : Inport  Port=4  OutDataTypeStr=fixdt(0, 12, 0)  PortDimensions=1  SampleTime=6.66666666666667e-09
  Simple Dual Port RAM : Subsystem
  rd_data : Outport
  wires:
  rd_addr/1 -> Simple Dual Port RAM/4(rd_addr)
  wr_en/1 -> Simple Dual Port RAM/3(wr_en)
  wr_addr/1 -> Simple Dual Port RAM/2(wr_addr)
  wr_data/1 -> Simple Dual Port RAM/1(wr_data)
  Simple Dual Port RAM/1(rd_data) -> rd_data/1

== system gm_parallel_lht/Parallel LHT/Parallel LHT Accumulator/Accumulator with Switches/Accumulator_instance135/Block RAM ==
  wr_data : Inport  OutDataTypeStr=fixdt(0, 12, 0)  PortDimensions=1  SampleTime=6.66666666666667e-09
  wr_addr : Inport  Port=2  OutDataTypeStr=fixdt(0, 12, 0)  PortDimensions=1  SampleTime=6.66666666666667e-09
  wr_en : Inport  Port=3  OutDataTypeStr=boolean  PortDimensions=1  SampleTime=6.66666666666667e-09
  rd_addr : Inport  Port=4  OutDataTypeStr=fixdt(0, 12, 0)  PortDimensions=1  SampleTime=6.66666666666667e-09
  Simple Dual Port RAM : Subsystem
  rd_data : Outport
  wires:
  rd_addr/1 -> Simple Dual Port RAM/4(rd_addr)
  wr_en/1 -> Simple Dual Port RAM/3(wr_en)
  wr_addr/1 -> Simple Dual Port RAM/2(wr_addr)
  wr_data/1 -> Simple Dual Port RAM/1(wr_data)
  Simple Dual Port RAM/1(rd_data) -> rd_data/1

== system gm_parallel_lht/Parallel LHT/Parallel LHT Accumulator/Accumulator with Switches/Accumulator_instance136/Block RAM ==
  wr_data : Inport  OutDataTypeStr=fixdt(0, 12, 0)  PortDimensions=1  SampleTime=6.66666666666667e-09
  wr_addr : Inport  Port=2  OutDataTypeStr=fixdt(0, 12, 0)  PortDimensions=1  SampleTime=6.66666666666667e-09
  wr_en : Inport  Port=3  OutDataTypeStr=boolean  PortDimensions=1  SampleTime=6.66666666666667e-09
  rd_addr : Inport  Port=4  OutDataTypeStr=fixdt(0, 12, 0)  PortDimensions=1  SampleTime=6.66666666666667e-09
  Simple Dual Port RAM : Subsystem
  rd_data : Outport
  wires:
  rd_addr/1 -> Simple Dual Port RAM/4(rd_addr)
  wr_en/1 -> Simple Dual Port RAM/3(wr_en)
  wr_addr/1 -> Simple Dual Port RAM/2(wr_addr)
  wr_data/1 -> Simple Dual Port RAM/1(wr_data)
  Simple Dual Port RAM/1(rd_data) -> rd_data/1

== system gm_parallel_lht/Parallel LHT/Parallel LHT Accumulator/Accumulator with Switches/Accumulator_instance137/Block RAM ==
  wr_data : Inport  OutDataTypeStr=fixdt(0, 12, 0)  PortDimensions=1  SampleTime=6.66666666666667e-09
  wr_addr : Inport  Port=2  OutDataTypeStr=fixdt(0, 12, 0)  PortDimensions=1  SampleTime=6.66666666666667e-09
  wr_en : Inport  Port=3  OutDataTypeStr=boolean  PortDimensions=1  SampleTime=6.66666666666667e-09
  rd_addr : Inport  Port=4  OutDataTypeStr=fixdt(0, 12, 0)  PortDimensions=1  SampleTime=6.66666666666667e-09
  Simple Dual Port RAM : Subsystem
  rd_data : Outport
  wires:
  rd_addr/1 -> Simple Dual Port RAM/4(rd_addr)
  wr_en/1 -> Simple Dual Port RAM/3(wr_en)
  wr_addr/1 -> Simple Dual Port RAM/2(wr_addr)
  wr_data/1 -> Simple Dual Port RAM/1(wr_data)
  Simple Dual Port RAM/1(rd_data) -> rd_data/1

== system gm_parallel_lht/Parallel LHT/Parallel LHT Accumulator/Accumulator with Switches/Accumulator_instance138/Block RAM ==
  wr_data : Inport  OutDataTypeStr=fixdt(0, 12, 0)  PortDimensions=1  SampleTime=6.66666666666667e-09
  wr_addr : Inport  Port=2  OutDataTypeStr=fixdt(0, 12, 0)  PortDimensions=1  SampleTime=6.66666666666667e-09
  wr_en : Inport  Port=3  OutDataTypeStr=boolean  PortDimensions=1  SampleTime=6.66666666666667e-09
  rd_addr : Inport  Port=4  OutDataTypeStr=fixdt(0, 12, 0)  PortDimensions=1  SampleTime=6.66666666666667e-09
  Simple Dual Port RAM : Subsystem
  rd_data : Outport
  wires:
  rd_addr/1 -> Simple Dual Port RAM/4(rd_addr)
  wr_en/1 -> Simple Dual Port RAM/3(wr_en)
  wr_addr/1 -> Simple Dual Port RAM/2(wr_addr)
  wr_data/1 -> Simple Dual Port RAM/1(wr_data)
  Simple Dual Port RAM/1(rd_data) -> rd_data/1

== system gm_parallel_lht/Parallel LHT/Parallel LHT Accumulator/Accumulator with Switches/Accumulator_instance139/Block RAM ==
  wr_data : Inport  OutDataTypeStr=fixdt(0, 12, 0)  PortDimensions=1  SampleTime=6.66666666666667e-09
  wr_addr : Inport  Port=2  OutDataTypeStr=fixdt(0, 12, 0)  PortDimensions=1  SampleTime=6.66666666666667e-09
  wr_en : Inport  Port=3  OutDataTypeStr=boolean  PortDimensions=1  SampleTime=6.66666666666667e-09
  rd_addr : Inport  Port=4  OutDataTypeStr=fixdt(0, 12, 0)  PortDimensions=1  SampleTime=6.66666666666667e-09
  Simple Dual Port RAM : Subsystem
  rd_data : Outport
  wires:
  rd_addr/1 -> Simple Dual Port RAM/4(rd_addr)
  wr_en/1 -> Simple Dual Port RAM/3(wr_en)
  wr_addr/1 -> Simple Dual Port RAM/2(wr_addr)
  wr_data/1 -> Simple Dual Port RAM/1(wr_data)
  Simple Dual Port RAM/1(rd_data) -> rd_data/1

== system gm_parallel_lht/Parallel LHT/Parallel LHT Accumulator/Accumulator with Switches/Accumulator_instance14/Block RAM ==
  wr_data : Inport  OutDataTypeStr=fixdt(0, 12, 0)  PortDimensions=1  SampleTime=6.66666666666667e-09
  wr_addr : Inport  Port=2  OutDataTypeStr=fixdt(0, 12, 0)  PortDimensions=1  SampleTime=6.66666666666667e-09
  wr_en : Inport  Port=3  OutDataTypeStr=boolean  PortDimensions=1  SampleTime=6.66666666666667e-09
  rd_addr : Inport  Port=4  OutDataTypeStr=fixdt(0, 12, 0)  PortDimensions=1  SampleTime=6.66666666666667e-09
  Simple Dual Port RAM : Subsystem
  rd_data : Outport
  wires:
  rd_addr/1 -> Simple Dual Port RAM/4(rd_addr)
  wr_en/1 -> Simple Dual Port RAM/3(wr_en)
  wr_addr/1 -> Simple Dual Port RAM/2(wr_addr)
  wr_data/1 -> Simple Dual Port RAM/1(wr_data)
  Simple Dual Port RAM/1(rd_data) -> rd_data/1

== system gm_parallel_lht/Parallel LHT/Parallel LHT Accumulator/Accumulator with Switches/Accumulator_instance140/Block RAM ==
  wr_data : Inport  OutDataTypeStr=fixdt(0, 12, 0)  PortDimensions=1  SampleTime=6.66666666666667e-09
  wr_addr : Inport  Port=2  OutDataTypeStr=fixdt(0, 12, 0)  PortDimensions=1  SampleTime=6.66666666666667e-09
  wr_en : Inport  Port=3  OutDataTypeStr=boolean  PortDimensions=1  SampleTime=6.66666666666667e-09
  rd_addr : Inport  Port=4  OutDataTypeStr=fixdt(0, 12, 0)  PortDimensions=1  SampleTime=6.66666666666667e-09
  Simple Dual Port RAM : Subsystem
  rd_data : Outport
  wires:
  rd_addr/1 -> Simple Dual Port RAM/4(rd_addr)
  wr_en/1 -> Simple Dual Port RAM/3(wr_en)
  wr_addr/1 -> Simple Dual Port RAM/2(wr_addr)
  wr_data/1 -> Simple Dual Port RAM/1(wr_data)
  Simple Dual Port RAM/1(rd_data) -> rd_data/1

== system gm_parallel_lht/Parallel LHT/Parallel LHT Accumulator/Accumulator with Switches/Accumulator_instance141/Block RAM ==
  wr_data : Inport  OutDataTypeStr=fixdt(0, 12, 0)  PortDimensions=1  SampleTime=6.66666666666667e-09
  wr_addr : Inport  Port=2  OutDataTypeStr=fixdt(0, 12, 0)  PortDimensions=1  SampleTime=6.66666666666667e-09
  wr_en : Inport  Port=3  OutDataTypeStr=boolean  PortDimensions=1  SampleTime=6.66666666666667e-09
  rd_addr : Inport  Port=4  OutDataTypeStr=fixdt(0, 12, 0)  PortDimensions=1  SampleTime=6.66666666666667e-09
  Simple Dual Port RAM : Subsystem
  rd_data : Outport
  wires:
  rd_addr/1 -> Simple Dual Port RAM/4(rd_addr)
  wr_en/1 -> Simple Dual Port RAM/3(wr_en)
  wr_addr/1 -> Simple Dual Port RAM/2(wr_addr)
  wr_data/1 -> Simple Dual Port RAM/1(wr_data)
  Simple Dual Port RAM/1(rd_data) -> rd_data/1

== system gm_parallel_lht/Parallel LHT/Parallel LHT Accumulator/Accumulator with Switches/Accumulator_instance142/Block RAM ==
  wr_data : Inport  OutDataTypeStr=fixdt(0, 12, 0)  PortDimensions=1  SampleTime=6.66666666666667e-09
  wr_addr : Inport  Port=2  OutDataTypeStr=fixdt(0, 12, 0)  PortDimensions=1  SampleTime=6.66666666666667e-09
  wr_en : Inport  Port=3  OutDataTypeStr=boolean  PortDimensions=1  SampleTime=6.66666666666667e-09
  rd_addr : Inport  Port=4  OutDataTypeStr=fixdt(0, 12, 0)  PortDimensions=1  SampleTime=6.66666666666667e-09
  Simple Dual Port RAM : Subsystem
  rd_data : Outport
  wires:
  rd_addr/1 -> Simple Dual Port RAM/4(rd_addr)
  wr_en/1 -> Simple Dual Port RAM/3(wr_en)
  wr_addr/1 -> Simple Dual Port RAM/2(wr_addr)
  wr_data/1 -> Simple Dual Port RAM/1(wr_data)
  Simple Dual Port RAM/1(rd_data) -> rd_data/1

== system gm_parallel_lht/Parallel LHT/Parallel LHT Accumulator/Accumulator with Switches/Accumulator_instance143/Block RAM ==
  wr_data : Inport  OutDataTypeStr=fixdt(0, 12, 0)  PortDimensions=1  SampleTime=6.66666666666667e-09
  wr_addr : Inport  Port=2  OutDataTypeStr=fixdt(0, 12, 0)  PortDimensions=1  SampleTime=6.66666666666667e-09
  wr_en : Inport  Port=3  OutDataTypeStr=boolean  PortDimensions=1  SampleTime=6.66666666666667e-09
  rd_addr : Inport  Port=4  OutDataTypeStr=fixdt(0, 12, 0)  PortDimensions=1  SampleTime=6.66666666666667e-09
  Simple Dual Port RAM : Subsystem
  rd_data : Outport
  wires:
  rd_addr/1 -> Simple Dual Port RAM/4(rd_addr)
  wr_en/1 -> Simple Dual Port RAM/3(wr_en)
  wr_addr/1 -> Simple Dual Port RAM/2(wr_addr)
  wr_data/1 -> Simple Dual Port RAM/1(wr_data)
  Simple Dual Port RAM/1(rd_data) -> rd_data/1

== system gm_parallel_lht/Parallel LHT/Parallel LHT Accumulator/Accumulator with Switches/Accumulator_instance144/Block RAM ==
  wr_data : Inport  OutDataTypeStr=fixdt(0, 12, 0)  PortDimensions=1  SampleTime=6.66666666666667e-09
  wr_addr : Inport  Port=2  OutDataTypeStr=fixdt(0, 12, 0)  PortDimensions=1  SampleTime=6.66666666666667e-09
  wr_en : Inport  Port=3  OutDataTypeStr=boolean  PortDimensions=1  SampleTime=6.66666666666667e-09
  rd_addr : Inport  Port=4  OutDataTypeStr=fixdt(0, 12, 0)  PortDimensions=1  SampleTime=6.66666666666667e-09
  Simple Dual Port RAM : Subsystem
  rd_data : Outport
  wires:
  rd_addr/1 -> Simple Dual Port RAM/4(rd_addr)
  wr_en/1 -> Simple Dual Port RAM/3(wr_en)
  wr_addr/1 -> Simple Dual Port RAM/2(wr_addr)
  wr_data/1 -> Simple Dual Port RAM/1(wr_data)
  Simple Dual Port RAM/1(rd_data) -> rd_data/1

== system gm_parallel_lht/Parallel LHT/Parallel LHT Accumulator/Accumulator with Switches/Accumulator_instance145/Block RAM ==
  wr_data : Inport  OutDataTypeStr=fixdt(0, 12, 0)  PortDimensions=1  SampleTime=6.66666666666667e-09
  wr_addr : Inport  Port=2  OutDataTypeStr=fixdt(0, 12, 0)  PortDimensions=1  SampleTime=6.66666666666667e-09
  wr_en : Inport  Port=3  OutDataTypeStr=boolean  PortDimensions=1  SampleTime=6.66666666666667e-09
  rd_addr : Inport  Port=4  OutDataTypeStr=fixdt(0, 12, 0)  PortDimensions=1  SampleTime=6.66666666666667e-09
  Simple Dual Port RAM : Subsystem
  rd_data : Outport
  wires:
  rd_addr/1 -> Simple Dual Port RAM/4(rd_addr)
  wr_en/1 -> Simple Dual Port RAM/3(wr_en)
  wr_addr/1 -> Simple Dual Port RAM/2(wr_addr)
  wr_data/1 -> Simple Dual Port RAM/1(wr_data)
  Simple Dual Port RAM/1(rd_data) -> rd_data/1

== system gm_parallel_lht/Parallel LHT/Parallel LHT Accumulator/Accumulator with Switches/Accumulator_instance146/Block RAM ==
  wr_data : Inport  OutDataTypeStr=fixdt(0, 12, 0)  PortDimensions=1  SampleTime=6.66666666666667e-09
  wr_addr : Inport  Port=2  OutDataTypeStr=fixdt(0, 12, 0)  PortDimensions=1  SampleTime=6.66666666666667e-09
  wr_en : Inport  Port=3  OutDataTypeStr=boolean  PortDimensions=1  SampleTime=6.66666666666667e-09
  rd_addr : Inport  Port=4  OutDataTypeStr=fixdt(0, 12, 0)  PortDimensions=1  SampleTime=6.66666666666667e-09
  Simple Dual Port RAM : Subsystem
  rd_data : Outport
  wires:
  rd_addr/1 -> Simple Dual Port RAM/4(rd_addr)
  wr_en/1 -> Simple Dual Port RAM/3(wr_en)
  wr_addr/1 -> Simple Dual Port RAM/2(wr_addr)
  wr_data/1 -> Simple Dual Port RAM/1(wr_data)
  Simple Dual Port RAM/1(rd_data) -> rd_data/1

== system gm_parallel_lht/Parallel LHT/Parallel LHT Accumulator/Accumulator with Switches/Accumulator_instance147/Block RAM ==
  wr_data : Inport  OutDataTypeStr=fixdt(0, 12, 0)  PortDimensions=1  SampleTime=6.66666666666667e-09
  wr_addr : Inport  Port=2  OutDataTypeStr=fixdt(0, 12, 0)  PortDimensions=1  SampleTime=6.66666666666667e-09
  wr_en : Inport  Port=3  OutDataTypeStr=boolean  PortDimensions=1  SampleTime=6.66666666666667e-09
  rd_addr : Inport  Port=4  OutDataTypeStr=fixdt(0, 12, 0)  PortDimensions=1  SampleTime=6.66666666666667e-09
  Simple Dual Port RAM : Subsystem
  rd_data : Outport
  wires:
  rd_addr/1 -> Simple Dual Port RAM/4(rd_addr)
  wr_en/1 -> Simple Dual Port RAM/3(wr_en)
  wr_addr/1 -> Simple Dual Port RAM/2(wr_addr)
  wr_data/1 -> Simple Dual Port RAM/1(wr_data)
  Simple Dual Port RAM/1(rd_data) -> rd_data/1

== system gm_parallel_lht/Parallel LHT/Parallel LHT Accumulator/Accumulator with Switches/Accumulator_instance148/Block RAM ==
  wr_data : Inport  OutDataTypeStr=fixdt(0, 12, 0)  PortDimensions=1  SampleTime=6.66666666666667e-09
  wr_addr : Inport  Port=2  OutDataTypeStr=fixdt(0, 12, 0)  PortDimensions=1  SampleTime=6.66666666666667e-09
  wr_en : Inport  Port=3  OutDataTypeStr=boolean  PortDimensions=1  SampleTime=6.66666666666667e-09
  rd_addr : Inport  Port=4  OutDataTypeStr=fixdt(0, 12, 0)  PortDimensions=1  SampleTime=6.66666666666667e-09
  Simple Dual Port RAM : Subsystem
  rd_data : Outport
  wires:
  rd_addr/1 -> Simple Dual Port RAM/4(rd_addr)
  wr_en/1 -> Simple Dual Port RAM/3(wr_en)
  wr_addr/1 -> Simple Dual Port RAM/2(wr_addr)
  wr_data/1 -> Simple Dual Port RAM/1(wr_data)
  Simple Dual Port RAM/1(rd_data) -> rd_data/1

== system gm_parallel_lht/Parallel LHT/Parallel LHT Accumulator/Accumulator with Switches/Accumulator_instance149/Block RAM ==
  wr_data : Inport  OutDataTypeStr=fixdt(0, 12, 0)  PortDimensions=1  SampleTime=6.66666666666667e-09
  wr_addr : Inport  Port=2  OutDataTypeStr=fixdt(0, 12, 0)  PortDimensions=1  SampleTime=6.66666666666667e-09
  wr_en : Inport  Port=3  OutDataTypeStr=boolean  PortDimensions=1  SampleTime=6.66666666666667e-09
  rd_addr : Inport  Port=4  OutDataTypeStr=fixdt(0, 12, 0)  PortDimensions=1  SampleTime=6.66666666666667e-09
  Simple Dual Port RAM : Subsystem
  rd_data : Outport
  wires:
  rd_addr/1 -> Simple Dual Port RAM/4(rd_addr)
  wr_en/1 -> Simple Dual Port RAM/3(wr_en)
  wr_addr/1 -> Simple Dual Port RAM/2(wr_addr)
  wr_data/1 -> Simple Dual Port RAM/1(wr_data)
  Simple Dual Port RAM/1(rd_data) -> rd_data/1

== system gm_parallel_lht/Parallel LHT/Parallel LHT Accumulator/Accumulator with Switches/Accumulator_instance15/Block RAM ==
  wr_data : Inport  OutDataTypeStr=fixdt(0, 12, 0)  PortDimensions=1  SampleTime=6.66666666666667e-09
  wr_addr : Inport  Port=2  OutDataTypeStr=fixdt(0, 12, 0)  PortDimensions=1  SampleTime=6.66666666666667e-09
  wr_en : Inport  Port=3  OutDataTypeStr=boolean  PortDimensions=1  SampleTime=6.66666666666667e-09
  rd_addr : Inport  Port=4  OutDataTypeStr=fixdt(0, 12, 0)  PortDimensions=1  SampleTime=6.66666666666667e-09
  Simple Dual Port RAM : Subsystem
  rd_data : Outport
  wires:
  rd_addr/1 -> Simple Dual Port RAM/4(rd_addr)
  wr_en/1 -> Simple Dual Port RAM/3(wr_en)
  wr_addr/1 -> Simple Dual Port RAM/2(wr_addr)
  wr_data/1 -> Simple Dual Port RAM/1(wr_data)
  Simple Dual Port RAM/1(rd_data) -> rd_data/1

== system gm_parallel_lht/Parallel LHT/Parallel LHT Accumulator/Accumulator with Switches/Accumulator_instance150/Block RAM ==
  wr_data : Inport  OutDataTypeStr=fixdt(0, 12, 0)  PortDimensions=1  SampleTime=6.66666666666667e-09
  wr_addr : Inport  Port=2  OutDataTypeStr=fixdt(0, 12, 0)  PortDimensions=1  SampleTime=6.66666666666667e-09
  wr_en : Inport  Port=3  OutDataTypeStr=boolean  PortDimensions=1  SampleTime=6.66666666666667e-09
  rd_addr : Inport  Port=4  OutDataTypeStr=fixdt(0, 12, 0)  PortDimensions=1  SampleTime=6.66666666666667e-09
  Simple Dual Port RAM : Subsystem
  rd_data : Outport
  wires:
  rd_addr/1 -> Simple Dual Port RAM/4(rd_addr)
  wr_en/1 -> Simple Dual Port RAM/3(wr_en)
  wr_addr/1 -> Simple Dual Port RAM/2(wr_addr)
  wr_data/1 -> Simple Dual Port RAM/1(wr_data)
  Simple Dual Port RAM/1(rd_data) -> rd_data/1
